simulink model "buck_converter_dcsource_output"  (R2023b)
settings: Solver=VariableStepAuto  StartTime=0.0  StopTime=0.012  RelTol=1e-3
libraries: spsDiodeLib x7, spsCurrentMeasurementLib x6, spsVoltageMeasurementLib x6, spsSeriesRLCBranchLib x4, spsACVoltageSourceLib x3, spsDCVoltageSourceLib x1, spsMosfetLib x1, spsPWMGeneratorDCDCLib x1, spspowerguiLib x1
settings Model: Creator=User  LastModifiedBy=User

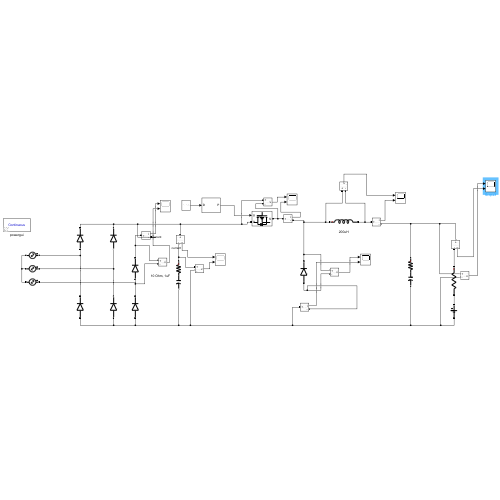
[thumbnail: Simulink's stored preview of the top-level diagram]
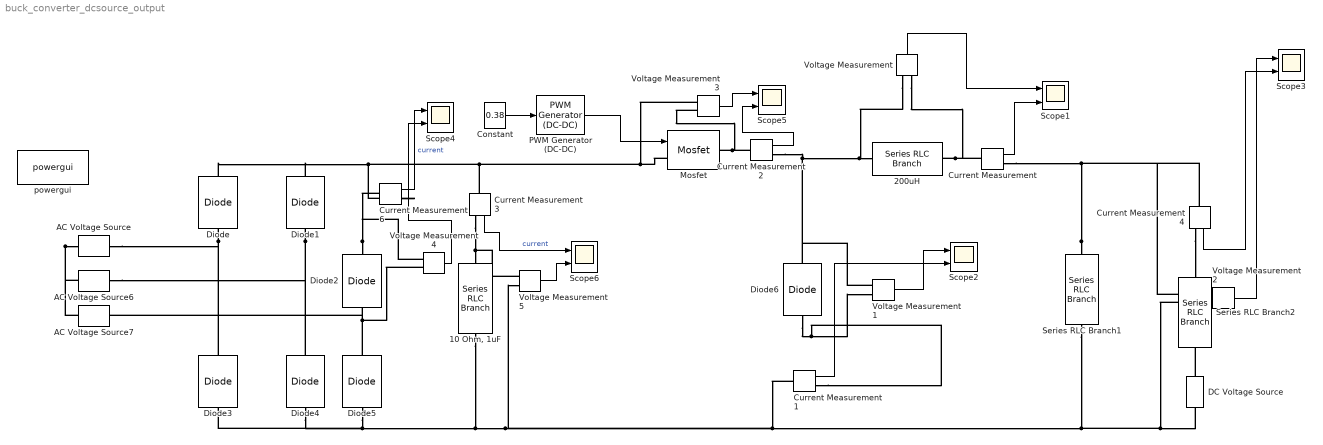
== system buck_converter_dcsource_output ==
  "10 Ohm, 1uF" : spsSeriesRLCBranchLib/Series RLC Branch  LConnTagsString=__new0  RConnTagsString=__new0  BranchType=RC  Resistance=10  Inductance=1e-3  SetiL0=off  InitialCurrent=0  Capacitance=1e-6  Setx0=off  InitialVoltage=50  Measurements=None
  200uH : spsSeriesRLCBranchLib/Series RLC Branch  LConnTagsString=__new0  RConnTagsString=__new0  BranchType=L  Resistance=1  Inductance=80e-6  SetiL0=off  InitialCurrent=0  Capacitance=1e-6  Setx0=off  InitialVoltage=0  Measurements=None
  AC Voltage Source : spsACVoltageSourceLib/AC Voltage Source  Amplitude=25*sqrt(2)/sqrt(3)  Phase=0  Frequency=50  SampleTime=0  Measurements=None  BusType=swing  Pref=10e3  Qref=0  Qmin=-inf  Qmax=+inf
  AC Voltage Source6 : spsACVoltageSourceLib/AC Voltage Source  Amplitude=25*sqrt(2)/sqrt(3)  Phase=120  Frequency=50  SampleTime=0  Measurements=None  BusType=swing  Pref=10e3  Qref=0  Qmin=-inf  Qmax=+inf
  AC Voltage Source7 : spsACVoltageSourceLib/AC Voltage Source  Amplitude=25*sqrt(2)/sqrt(3)  Phase=240  Frequency=50  SampleTime=0  Measurements=None  BusType=swing  Pref=10e3  Qref=0  Qmin=-inf  Qmax=+inf
  Constant : Constant  Value=0.38
  Current Measurement{,1..4,6} (6 alike) : spsCurrentMeasurementLib/Current Measurement  PhasorSimulation=off  OutputType=Complex  PSBequivalent=0
  DC Voltage Source : spsDCVoltageSourceLib/DC Voltage Source  Amplitude=10.5  Measurements=Voltage
  Diode{,1..6} (7 alike) : spsDiodeLib/Diode  Ron=0.001  Lon=0  Vf=0.8  IC=0  UseSnubber=0  Rs=0  Cs=0  Measurements=off
  Mosfet : spsMosfetLib/Mosfet  Ron=0.1  Lon=0  Rd=0.01  Vfd=0  IC=0  Rs=1e5  Cs=inf  Measurements=off
  PWM Generator (DC-DC) : spsPWMGeneratorDCDCLib/PWM Generator (DC-DC)  Fsw=50000  Ts=0
  Scope{1..6} (6 alike) : Scope  NumInputPorts=2
  Series RLC Branch1 : spsSeriesRLCBranchLib/Series RLC Branch  LConnTagsString=__new0  RConnTagsString=__new0  BranchType=RC  Resistance=0.0025  Inductance=1e-3  SetiL0=off  InitialCurrent=0  Capacitance=22e-6  Setx0=off  InitialVoltage=0  Measurements=None
  Series RLC Branch2 : spsSeriesRLCBranchLib/Series RLC Branch  LConnTagsString=__new0  RConnTagsString=__new0  BranchType=R  Resistance=0.1  Inductance=1e-3  SetiL0=off  InitialCurrent=0  Capacitance=1e-6  Setx0=off  InitialVoltage=0  Measurements=None
  Voltage Measurement{,1..5} (6 alike) : spsVoltageMeasurementLib/Voltage Measurement  PhasorSimulation=off  OutputType=Complex  PSBequivalent=0
  powergui : spspowerguiLib/powergui  Priority=1  SimulationMode=Continuous  SampleTime=0.0002  frequency=60  Iterations=50  frequencyindice=0  Pbase=100e6  ErrMax=1e-4  UnitsV=kV  UnitsW=MW  buscounter=0  FunctionMessages=off  echomessages=off  EnableUseOfTLC=off  CurrentSourceSwitches=off  DisableSnubberDevices=off  DisableRonSwitches=off  DisableVfSwitches=off  DisplayEquations=off  AutomaticDiscreteSolvers=off  SolverType=Tustin/Backward Euler (TBE)  Interpol=off  ExternalGateDelay=off  methode=off  Ts=100  x0status=blocks  SPID=on  SwTol=0  HookPort=off  NonlinearTolerance=1e-4  nMaxIteration=100  ContinueOnMaxIteration=off  RestoreLinks=warning  ResistiveCurrentMeasurement=off  Frange=[0:2:500]  Ylog=off  Xlog=on  ShowGrid=off  save=off  variable=ZData  structure=0  ZoomFFT=off  StartTime=0.0  cycles=1  DisplayStyle=1  fundamental=60  FreqAxis=off  MaxFrequency=1000  frequencyindicesteady=1  RmsSteady=1  display=off
  wires:
  Constant/1 -> PWM Generator (DC-DC)/1
  Current Measurement2/1 -> Scope5/2
  Voltage Measurement4/1 -> Scope4/2
  Voltage Measurement3/1 -> Scope5/1
  Current Measurement6/1 -> Scope4/1  "current"
  Voltage Measurement5/1 -> Scope6/2
  Voltage Measurement2/1 -> Scope3/1
  Current Measurement3/1 -> Scope6/1  "current"
  Current Measurement/1 -> Scope1/2
  Voltage Measurement/1 -> Scope1/1
  Current Measurement1/1 -> Scope2/2
  Voltage Measurement1/1 -> Scope2/1
  PWM Generator (DC-DC)/1 -> Mosfet/1
  Current Measurement4/1 -> Scope3/2
  connections:
  Voltage Measurement2/LConn2 -- DC Voltage Source/LConn1 -- Series RLC Branch1/RConn1 -- Current Measurement1/LConn1 -- Voltage Measurement5/LConn2 -- "10 Ohm, 1uF"/RConn1 -- Diode5/LConn1 -- Diode4/LConn1 -- Diode3/LConn1
  "10 Ohm, 1uF"/LConn1 -- Voltage Measurement5/LConn1 -- Current Measurement3/RConn1
  Mosfet/RConn1 -- Current Measurement2/LConn1 -- Voltage Measurement3/LConn2
  Diode1/LConn1 -- Diode4/RConn1 -- AC Voltage Source6/RConn1
  Diode2/LConn1 -- Diode5/RConn1 -- Voltage Measurement4/LConn2 -- AC Voltage Source7/RConn1
  Current Measurement1/RConn1 -- Diode6/LConn1 -- Voltage Measurement1/LConn2
  Mosfet/LConn1 -- Diode/RConn1 -- Diode1/RConn1 -- Current Measurement6/RConn1 -- Current Measurement3/LConn1 -- Voltage Measurement3/LConn1
  Diode2/RConn1 -- Current Measurement6/LConn1 -- Voltage Measurement4/LConn1
  200uH/RConn1 -- Voltage Measurement/LConn2 -- Current Measurement/LConn1
  Series RLC Branch1/LConn1 -- Current Measurement/RConn1 -- Current Measurement4/LConn1 -- Voltage Measurement2/LConn1
  200uH/LConn1 -- Voltage Measurement/LConn1 -- Voltage Measurement1/LConn1 -- Diode6/RConn1 -- Current Measurement2/RConn1
  AC Voltage Source/LConn1 -- AC Voltage Source7/LConn1 -- AC Voltage Source6/LConn1
  Diode/LConn1 -- Diode3/RConn1 -- AC Voltage Source/RConn1
  DC Voltage Source/RConn1 -- Series RLC Branch2/RConn1
  Current Measurement4/RConn1 -- Series RLC Branch2/LConn1
